simulink model "boat_model_and_controller2020mpc"  (R2020b)
settings: Solver=VariableStepAuto  StartTime=0.0  StopTime=10  FixedStep=0.01  RelTol=1e-3
undefined symbols (not defined in the file): DiscIntNeverNeededParam, Eff, FF_L, FF_R, initial_P, initial_Pitch, initial_Q, initial_R, initial_ROLL, initial_uspeed, initial_vspeed, initial_wspeed, initial_YAW, initial_Z, Kih, Kir, rear_alfas, T, uncertainty
libraries: simulink x7, simulink_extras x3, dspsrcs4 x1, mpclib x1, pid_lib x1
(part 1 of 3)
settings Model: Creator=Basile  LastModifiedBy=sasas
settings SolverCC: ConcurrentTasks=on  PositivePriorityOrder=on
settings DataIOCC: ExternalInput=getinputstruct(op_trim1)  InitialState=getstatestruct(op_trim1)  SaveOutput=off  DSMLogging=off  SaveTime=off  ReturnWorkspaceOutputs=off
settings OptimizationCC: BlockReduction=off  DefaultParameterBehavior=Inlined  UseDivisionForNetSlopeComputation=on  UseFloatMulNetSlope=on  OptimizeBlockIOStorage=off  BufferReuse=off  PassReuseOutputArgsThreshold=0  EfficientFloat2IntCast=on  OptimizeBlockOrder=speed  DifferentSizesBufferReuse=on
settings DebuggingCC: InheritedTsInSrcMsg=none  ParameterTunabilityLossMsg=error  UnconnectedInputMsg=none  UnconnectedOutputMsg=none  UnconnectedLineMsg=none  UniqueDataStoreMsg=error  ArithmeticOperatorsInVariantConditions=warning
settings HardwareCC: ProdBitPerLong=64  ProdLongLongMode=on  ProdHWDeviceType=Intel->x86-64 (Linux 64)
settings SFSimCC: SimUseLocalCustomCode=off  MATLABDynamicMemAlloc=off  CustomCodeUndefinedFunction=UseInterfaceOnly
settings RTWCC: Description=Simulink Real-Time  SystemTargetFile=slrealtime.tlc  TemplateMakefile=slrealtime_default_tmf  GenerateReport=on  RTWUseLocalCustomCode=off  Toolchain=Simulink Real-Time Toolchain  BuildConfiguration=Faster Runs  LaunchReport=on  CodeExecutionProfiling=on  TargetLang=C++
settings CodeAppCC: ForceParamTrailComments=on  OperatorAnnotations=on

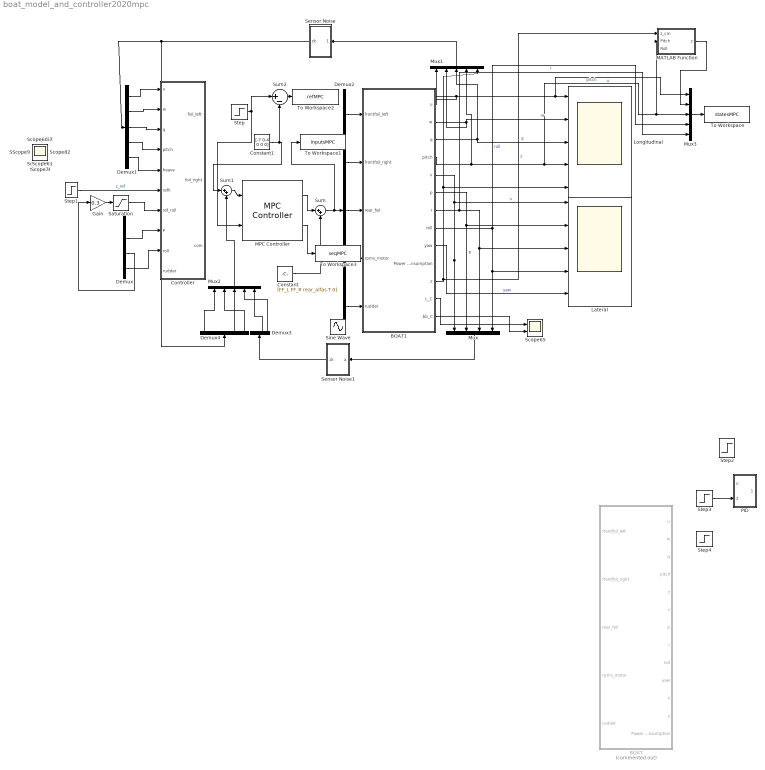
== system boat_model_and_controller2020mpc ==
  BOAT : Subsystem  Commented=on
  BOAT1 : Subsystem
  Constant : Constant  Value=[FF_L FF_R rear_alfas T 0]
  Constant1 : Constant  Value=[-7 0.4 0 0 0]
  Controller : Subsystem
  Demux : Demux
  Demux1 : Demux  Outputs=5
  Demux2 : Demux  Outputs=5
  Demux3 : Demux
  Demux4 : Demux  Outputs=5
  Gain : Gain  Gain=0.3
  Lateral : Scope  NumInputPorts=5
  Longitudinal : Scope  NumInputPorts=5
  MATLAB Function : MATLAB Function  TreatAsAtomicUnit=on
  MPC Controller : mpclib/MPC Controller  SCDEnableBlockLinearizationSpecification=on  mpcobj=mpcobj  x0=Boat_mpc  is_multiple=0  enable_value=0  return_u0=off  updateMPCinCallerWorkspace=on  md_inport=off  mv_inport=off  uref_inport=off  return_cost=off  return_mvseq=off  return_qpstatus=off  return_xseq=off  return_state=off  return_ovseq=on  state_inport=off  umin_inport=off  umax_inport=off  ymin_inport=off  ymax_inport=off  cc_inport=off  ywt_inport=off  uwt_inport=off  duwt_inport=off  rhoeps_inport=off  pm_inport=off  MaximumP=10  HorizonChoice=FixedHorizon  n_ts=0.1  n_p=20  n_mv=5  n_md=0  n_ud=0  n_mo=5  n_uo=0  BlockDataType=double  SampleTimeInherited=off  switch_inport=off
  Mux : Mux
  Mux1 : Mux  Inputs=5
  Mux2 : Mux  Inputs=5
  Mux3 : Mux  Inputs=5
  PID : Subsystem
  Saturation : Saturate  UpperLimit=3  LowerLimit=-3
  Scope65 : Scope  NumInputPorts=2
  Sensor Noise : Subsystem
  Sensor Noise1 : Subsystem
  Sine Wave : Sin  Amplitude=15  Frequency=0.1*2*pi  SampleTime=0
  Step : Step  Before=[0 0 0 0 0]  After=[1 -0.1 1 1 1]  SampleTime=0
  Step1 : Step  Time=0  Before=initial_Z  After=initial_Z  SampleTime=0
  Step2 : Step  Time=0  Before=rear_alfas  After=rear_alfas  SampleTime=0
  Step3 : Step  Time=10  Before=initial_uspeed  After=8  SampleTime=0
  Step4 : Step  Time=0  Before=15  After=15  SampleTime=0
  Sum : Sum  Inputs=|++
  Sum1 : Sum  Inputs=|++
  Sum2 : Sum  Inputs=|+-
  To Workspace : ToWorkspace  VariableName=statesMPC  SaveFormat=Timeseries  SampleTime=-1
  To Workspace1 : ToWorkspace  VariableName=inputsMPC  SaveFormat=Timeseries  SampleTime=-1
  To Workspace2 : ToWorkspace  VariableName=refMPC  SaveFormat=Timeseries  SampleTime=-1
  To Workspace3 : ToWorkspace  VariableName=seqMPC  SaveFormat=Timeseries  SampleTime=-1
  Scope{,1..64} (65 alike) : Scope
  wires:
  BOAT1/2(w) -> Longitudinal/2, Mux1/2  "w"
  BOAT1/3(q) -> Longitudinal/3, Mux1/3  "q"
  BOAT1/5(v) -> Mux/1, Lateral/1  "v"
  BOAT1/6(p) -> Mux/2, Lateral/2  "p"
  BOAT1/8(roll) -> Mux/4, Lateral/4, Mux3/4  "roll"
  BOAT1/11(z) -> MATLAB Function/1(z_cm), Mux1/5, Longitudinal/5  "z"
  BOAT1/1(u) -> Mux3/1, Longitudinal/1, Mux1/1  "u"
  BOAT1/7(r) -> Mux3/5, Mux/3, Lateral/3  "r"
  Demux/2 -> Controller/8(P)
  Demux1/2 -> Controller/2(w)
  Demux1/3 -> Controller/3(q)
  Demux1/4 -> Controller/4(pitch)
  Demux1/5 -> Controller/5(heave)
  Demux1/1 -> Controller/1(u)
  BOAT1/9(yaw) -> Lateral/5  "yaw"
  BOAT1/4(pitch) -> MATLAB Function/2(Pitch), Mux3/3, Longitudinal/4, Mux1/4  "pitch"
  Demux/4 -> Controller/9(roll)
  Mux1/1 -> Sensor Noise/1(states)
  Step1/1 -> Controller/6(refh)  "z_ref"
  Mux/1 -> Sensor Noise1/1(a)
  Step3/1 -> PID/2(In2)
  Gain/1 -> Saturation/1
  Saturation/1 -> Controller/7(ref_roll)
  Demux/3 -> Gain/1
  BOAT1/12(L_C) -> Scope65/1
  BOAT1/13(bb_C) -> Scope65/2
  Demux2/1 -> BOAT1/1(frontfoil_left)
  Demux2/2 -> BOAT1/2(frontfoil_right)
  Demux2/3 -> BOAT1/3(rear_foil)
  Demux2/4 -> BOAT1/4(rpms_motor)
  Demux2/5 -> BOAT1/5(rudder)
  MPC Controller/1 -> Sum/1
  Sensor Noise1/1(zk) -> Demux3/1
  Demux4/1 -> Mux2/1
  Demux4/5 -> Mux2/2
  Demux4/4 -> Mux2/3
  Demux3/4 -> Mux2/4
  Demux3/3 -> Mux2/5
  Sum1/1 -> MPC Controller/1
  Mux2/1 -> Sum1/2
  Constant1/1 -> Sum1/1, Sum2/2
  Step/1 -> MPC Controller/2, Sum2/1
  Sensor Noise/1(zk) -> Demux1/1, Demux4/1
  Sum/1 -> To Workspace1/1, Demux2/1
  Constant/1 -> Sum/2
  Mux3/1 -> To Workspace/1
  Sum2/1 -> To Workspace2/1
  MATLAB Function/1(z) -> Mux3/2
  MPC Controller/2 -> To Workspace3/1

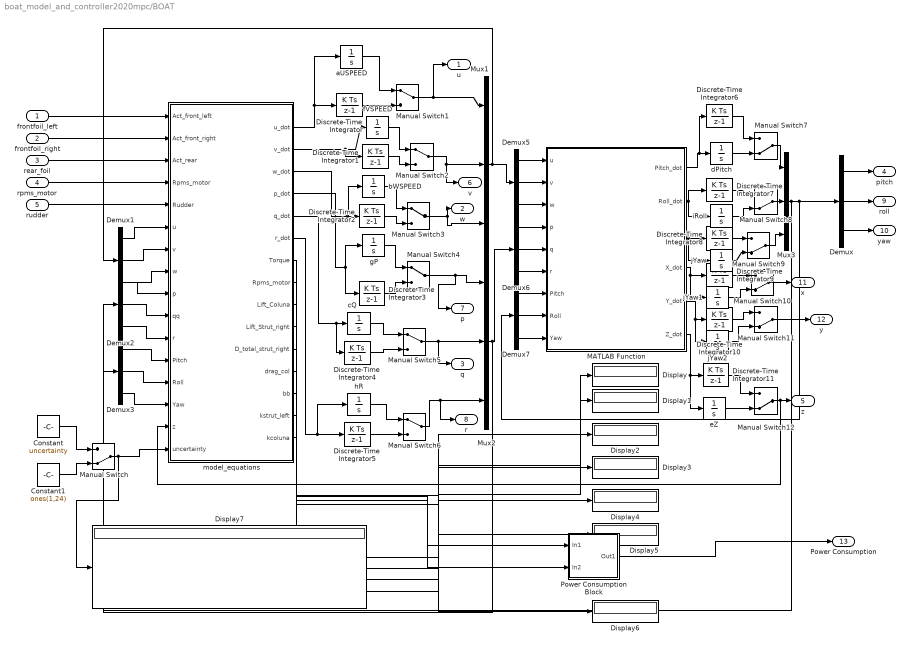
== system boat_model_and_controller2020mpc/BOAT ==
  frontfoil_left : Inport
  frontfoil_right : Inport  Port=2
  rear_foil : Inport  Port=3
  rpms_motor : Inport  Port=4
  rudder : Inport  Port=5
  Constant : Constant  Value=uncertainty
  Constant1 : Constant  Value=ones(1,24)
  Demux{,1..3,5..7} (7 alike) : Demux  Outputs=3
  Discrete-Time Integrator : DiscreteIntegrator  InitialCondition=initial_uspeed  SampleTime=-1  ICPrevOutput=DiscIntNeverNeededParam  ICPrevScaledInput=DiscIntNeverNeededParam
  Discrete-Time Integrator{1..10} (10 alike) : DiscreteIntegrator  SampleTime=-1  ICPrevOutput=DiscIntNeverNeededParam  ICPrevScaledInput=DiscIntNeverNeededParam
  Discrete-Time Integrator11 : DiscreteIntegrator  InitialCondition=initial_Z  SampleTime=-1  ICPrevOutput=DiscIntNeverNeededParam  ICPrevScaledInput=DiscIntNeverNeededParam
  Display{,1..7} (8 alike) : Display
  MATLAB Function : MATLAB Function  TreatAsAtomicUnit=on
  Manual Switch{,7..12} (7 alike) : ManualSwitch  CurrentSetting=0
  Manual Switch{1..6} (6 alike) : ManualSwitch
  Mux1 : Mux  Inputs=3
  Mux2 : Mux  Inputs=3
  Mux3 : Mux  Inputs=3
  Power Consumption Block : Subsystem
  aUSPEED : Integrator  InitialCondition=initial_uspeed
  bWSPEED : Integrator  InitialCondition=initial_wspeed
  cQ : Integrator  InitialCondition=initial_Q
  dPitch : Integrator  InitialCondition=initial_Pitch
  eZ : Integrator  InitialCondition=initial_Z
  fVSPEED : Integrator  InitialCondition=initial_vspeed
  gP : Integrator  InitialCondition=initial_P
  hR : Integrator  InitialCondition=initial_R
  iRoll : Integrator  InitialCondition=initial_ROLL
  jYaw : Integrator  InitialCondition=initial_YAW
  jYaw1 : Integrator
  jYaw2 : Integrator
  model_equations : MATLAB Function  TreatAsAtomicUnit=on  VariantControl=Variant1
  u : Outport  VectorParamsAs1DForOutWhenUnconnected=off
  w : Outport  Port=2  VectorParamsAs1DForOutWhenUnconnected=off
  q : Outport  Port=3  VectorParamsAs1DForOutWhenUnconnected=off
  pitch : Outport  Port=4  VectorParamsAs1DForOutWhenUnconnected=off
  z : Outport  Port=5  VectorParamsAs1DForOutWhenUnconnected=off
  v : Outport  Port=6  VectorParamsAs1DForOutWhenUnconnected=off
  p : Outport  Port=7  VectorParamsAs1DForOutWhenUnconnected=off
  r : Outport  Port=8  VectorParamsAs1DForOutWhenUnconnected=off
  roll : Outport  Port=9  VectorParamsAs1DForOutWhenUnconnected=off
  yaw : Outport  Port=10  VectorParamsAs1DForOutWhenUnconnected=off
  x : Outport  Port=11  VectorParamsAs1DForOutWhenUnconnected=off
  y : Outport  Port=12  VectorParamsAs1DForOutWhenUnconnected=off
  Power Consumption : Outport  Port=13  VectorParamsAs1DForOutWhenUnconnected=off
  wires:
  model_equations/6(r_dot) -> hR/1, Discrete-Time Integrator5/1
  Demux5/3 -> MATLAB Function/3(w)
  frontfoil_left/1 -> model_equations/1(Act_front_left)
  frontfoil_right/1 -> model_equations/2(Act_front_right)
  Mux1/1 -> Demux5/1, Demux1/1
  Demux/2 -> roll/1
  Demux7/2 -> MATLAB Function/8(Roll)
  Demux7/3 -> MATLAB Function/9(Yaw)
  model_equations/5(q_dot) -> Discrete-Time Integrator4/1, cQ/1
  rear_foil/1 -> model_equations/3(Act_rear)
  model_equations/3(w_dot) -> bWSPEED/1, Discrete-Time Integrator2/1
  Demux3/2 -> model_equations/13(Roll)
  Demux2/2 -> model_equations/10(qq)
  Demux2/3 -> model_equations/11(r)
  model_equations/4(p_dot) -> Discrete-Time Integrator3/1, gP/1
  Demux2/1 -> model_equations/9(p)
  Demux5/1 -> MATLAB Function/1(u)
  rpms_motor/1 -> model_equations/4("Rpms_motor ")
  MATLAB Function/2(Roll_dot) -> iRoll/1, Discrete-Time Integrator7/1
  Demux7/1 -> MATLAB Function/7(Pitch)
  Mux3/1 -> Demux/1, Demux7/1, Demux3/1
  Demux3/1 -> model_equations/12(Pitch)
  model_equations/2(v_dot) -> fVSPEED/1, Discrete-Time Integrator1/1
  Demux/1 -> pitch/1
  Demux1/2 -> model_equations/7(v)
  Demux6/1 -> MATLAB Function/4(p)
  MATLAB Function/1(Pitch_dot) -> Discrete-Time Integrator6/1, dPitch/1
  Mux2/1 -> Demux6/1, Demux2/1
  Demux5/2 -> MATLAB Function/2(v)
  Demux/3 -> yaw/1
  rudder/1 -> model_equations/5(Rudder)
  Demux6/2 -> MATLAB Function/5(q)
  Demux1/3 -> model_equations/8(w)
  Demux6/3 -> MATLAB Function/6(r)
  Demux3/3 -> model_equations/14(Yaw)
  MATLAB Function/5(Y_dot) -> Discrete-Time Integrator10/1, jYaw2/1
  MATLAB Function/4(X_dot) -> Discrete-Time Integrator9/1, jYaw1/1
  model_equations/8(Rpms_motor) -> Power Consumption Block/2(In2)
  Power Consumption Block/1(Out1) -> Power Consumption/1
  model_equations/7(Torque) -> Power Consumption Block/1(In1)
  model_equations/9(Lift_Coluna) -> Display/1
  model_equations/10(Lift_Strut_right) -> Display1/1
  model_equations/11(D_total_strut_right) -> Display2/1
  model_equations/12(drag_col) -> Display3/1
  model_equations/13(bb) -> Display4/1
  model_equations/14(kstrut_left) -> Display5/1
  model_equations/15(kcoluna) -> Display6/1
  Demux1/1 -> model_equations/6(u)
  Constant/1 -> Manual Switch/1
  Manual Switch/1 -> model_equations/16(uncertainty), Display7/1
  Constant1/1 -> Manual Switch/2
  Discrete-Time Integrator/1 -> Manual Switch1/2
  Manual Switch1/1 -> Mux1/1, u/1
  aUSPEED/1 -> Manual Switch1/1
  fVSPEED/1 -> Manual Switch2/1
  Manual Switch2/1 -> v/1, Mux1/2
  bWSPEED/1 -> Manual Switch3/1
  Manual Switch3/1 -> Mux1/3, w/1
  gP/1 -> Manual Switch4/1
  Manual Switch4/1 -> Mux2/1, p/1
  cQ/1 -> Manual Switch5/1
  Manual Switch5/1 -> Mux2/2, q/1
  Manual Switch6/1 -> r/1, Mux2/3
  hR/1 -> Manual Switch6/1
  Discrete-Time Integrator1/1 -> Manual Switch2/2
  Discrete-Time Integrator2/1 -> Manual Switch3/2
  Discrete-Time Integrator3/1 -> Manual Switch4/2
  Discrete-Time Integrator4/1 -> Manual Switch5/2
  Discrete-Time Integrator5/1 -> Manual Switch6/2
  Manual Switch7/1 -> Mux3/1
  dPitch/1 -> Manual Switch7/2
  Discrete-Time Integrator6/1 -> Manual Switch7/1
  Manual Switch8/1 -> Mux3/2
  iRoll/1 -> Manual Switch8/2
  Discrete-Time Integrator7/1 -> Manual Switch8/1
  Manual Switch9/1 -> Mux3/3
  jYaw/1 -> Manual Switch9/2
  Discrete-Time Integrator8/1 -> Manual Switch9/1
  MATLAB Function/3(Yaw_dot) -> Discrete-Time Integrator8/1, jYaw/1
  Manual Switch10/1 -> x/1
  jYaw1/1 -> Manual Switch10/2
  Discrete-Time Integrator9/1 -> Manual Switch10/1
  Manual Switch11/1 -> y/1
  Discrete-Time Integrator10/1 -> Manual Switch11/1
  jYaw2/1 -> Manual Switch11/2
  Manual Switch12/1 -> model_equations/15(z), z/1
  eZ/1 -> Manual Switch12/2
  Discrete-Time Integrator11/1 -> Manual Switch12/1
  MATLAB Function/6(Z_dot) -> eZ/1, Discrete-Time Integrator11/1
  model_equations/1(u_dot) -> aUSPEED/1, Discrete-Time Integrator/1

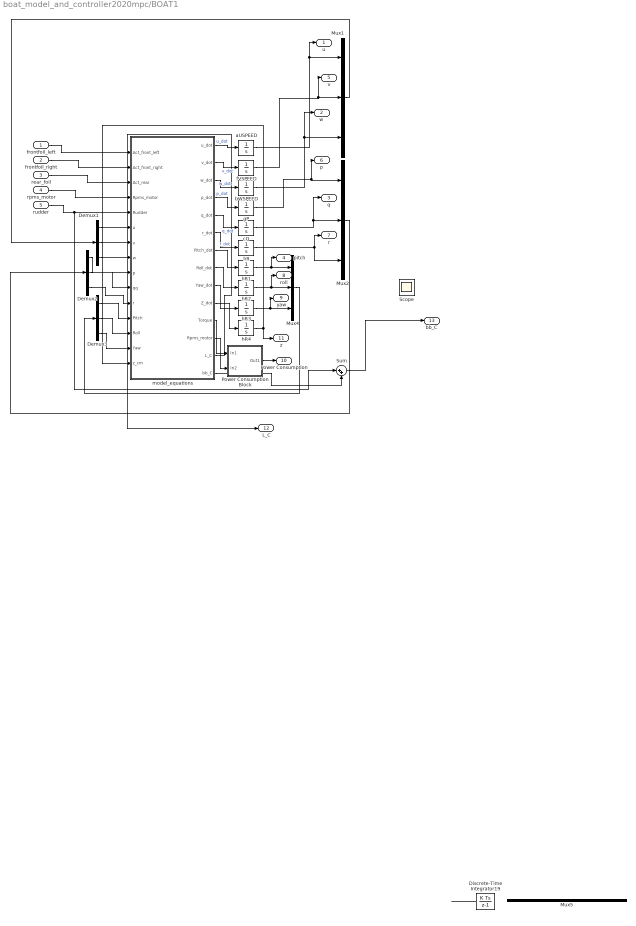
== system boat_model_and_controller2020mpc/BOAT1 ==
  frontfoil_left : Inport
  frontfoil_right : Inport  Port=2
  rear_foil : Inport  Port=3
  rpms_motor : Inport  Port=4
  rudder : Inport  Port=5
  Demux1 : Demux  Outputs=3
  Demux2 : Demux  Outputs=3
  Demux3 : Demux  Outputs=3
  Discrete-Time Integrator19 : DiscreteIntegrator  InitialCondition=-0.4  SampleTime=-1  ICPrevOutput=DiscIntNeverNeededParam  ICPrevScaledInput=DiscIntNeverNeededParam
  Mux{1..2,4..5} (4 alike) : Mux  Inputs=3
  Power Consumption Block : Subsystem
  Scope : Scope
  Sum : Sum  Inputs=|++
  aUSPEED : Integrator  InitialCondition=initial_uspeed
  bWSPEED : Integrator  InitialCondition=initial_wspeed
  cQ : Integrator  InitialCondition=initial_Q
  fVSPEED : Integrator  InitialCondition=initial_vspeed
  gP : Integrator  InitialCondition=initial_P
  hR : Integrator  InitialCondition=initial_R
  hR1 : Integrator
  hR2 : Integrator
  hR3 : Integrator
  hR4 : Integrator  InitialCondition=initial_Z
  model_equations : MATLAB Function  TreatAsAtomicUnit=on  VariantControl=Variant1
  u : Outport  VectorParamsAs1DForOutWhenUnconnected=off
  w : Outport  Port=2  VectorParamsAs1DForOutWhenUnconnected=off
  q : Outport  Port=3  VectorParamsAs1DForOutWhenUnconnected=off
  pitch : Outport  Port=4  VectorParamsAs1DForOutWhenUnconnected=off
  v : Outport  Port=5  VectorParamsAs1DForOutWhenUnconnected=off
  p : Outport  Port=6  VectorParamsAs1DForOutWhenUnconnected=off
  r : Outport  Port=7  VectorParamsAs1DForOutWhenUnconnected=off
  roll : Outport  Port=8  VectorParamsAs1DForOutWhenUnconnected=off
  yaw : Outport  Port=9  VectorParamsAs1DForOutWhenUnconnected=off
  Power Consumption : Outport  Port=10  VectorParamsAs1DForOutWhenUnconnected=off
  z : Outport  Port=11  VectorParamsAs1DForOutWhenUnconnected=off
  L_C : Outport  Port=12  VectorParamsAs1DForOutWhenUnconnected=off
  bb_C : Outport  Port=13  VectorParamsAs1DForOutWhenUnconnected=off
  wires:
  model_equations/6(r_dot) -> hR/1  "r_dot"
  Mux1/1 -> Demux1/1
  model_equations/5(q_dot) -> cQ/1  "q_dot"
  rear_foil/1 -> model_equations/3(Act_rear)
  Demux3/2 -> model_equations/13(Roll)
  Demux2/2 -> model_equations/10(qq)
  Demux2/3 -> model_equations/11(r)
  model_equations/4(p_dot) -> gP/1  "p_dot"
  Demux2/1 -> model_equations/9(p)
  rpms_motor/1 -> model_equations/4("Rpms_motor ")
  Demux3/1 -> model_equations/12(Pitch)
  model_equations/2(v_dot) -> fVSPEED/1  "v_dot"
  Demux1/2 -> model_equations/7(v)
  Mux2/1 -> Demux2/1
  Demux1/3 -> model_equations/8(w)
  Demux3/3 -> model_equations/14(Yaw)
  model_equations/12(Rpms_motor) -> Power Consumption Block/2(In2)
  Power Consumption Block/1(Out1) -> Power Consumption/1
  model_equations/11(Torque) -> Power Consumption Block/1(In1)
  Demux1/1 -> model_equations/6(u)
  aUSPEED/1 -> u/1, Mux1/1
  fVSPEED/1 -> v/1, Mux1/2
  cQ/1 -> q/1, Mux2/2
  hR/1 -> Mux2/3, r/1
  model_equations/3(w_dot) -> bWSPEED/1  "w_dot"
  model_equations/1(u_dot) -> aUSPEED/1  "u_dot"
  Discrete-Time Integrator19/1 -> ?
  bWSPEED/1 -> w/1, Mux1/3
  gP/1 -> p/1, Mux2/1
  model_equations/10(Z_dot) -> hR4/1
  model_equations/7(Pitch_dot) -> hR1/1
  model_equations/8(Roll_dot) -> hR2/1
  model_equations/9(Yaw_dot) -> hR3/1
  hR1/1 -> pitch/1, Mux4/1
  hR2/1 -> roll/1, Mux4/2
  hR3/1 -> yaw/1, Mux4/3
  Mux4/1 -> Demux3/1
  hR4/1 -> z/1, model_equations/15(z_cm)
  model_equations/13(L_C) -> L_C/1
  rudder/1 -> Sum/1, model_equations/5(Rudder)
  model_equations/14(bb_C) -> Sum/2
  Sum/1 -> bb_C/1
  frontfoil_left/1 -> model_equations/1(Act_front_left)
  frontfoil_right/1 -> model_equations/2(Act_front_right)

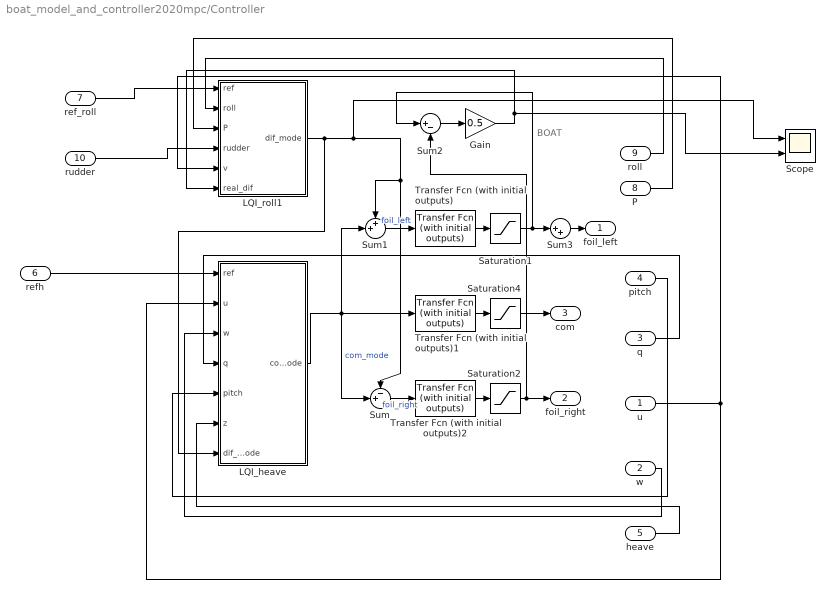
== system boat_model_and_controller2020mpc/Controller ==
  note: BOAT
  u : Inport
  w : Inport  Port=2
  q : Inport  Port=3
  pitch : Inport  Port=4
  heave : Inport  Port=5
  refh : Inport  Port=6
  ref_roll : Inport  Port=7
  P : Inport  Port=8
  roll : Inport  Port=9
  rudder : Inport  Port=10
  Gain : Gain  Gain=0.5
  LQI_heave : Subsystem  TreatAsAtomicUnit=on  SystemSampleTime=0.02
      settings: MinAlgLoopOccurrences=on
  LQI_roll1 : Subsystem  TreatAsAtomicUnit=on  SystemSampleTime=0.02
  Saturation1 : Saturate  UpperLimit=14  LowerLimit=-3
  Saturation2 : Saturate  UpperLimit=14  LowerLimit=-3
  Saturation4 : Saturate  UpperLimit=14  LowerLimit=-3
  Scope : Scope  NumInputPorts=2
  Sum : Sum  Inputs=-+|
  Sum1 : Sum  Inputs=++|
  Sum2 : Sum  Inputs=|+-
  Sum3 : Sum  Inputs=|++
  Transfer Fcn (with initial outputs) : simulink_extras/Additional Linear/Transfer Fcn (with initial outputs)  N=[40]  D="[1  40]"  Y0=FF_L  U0=FF_L
  Transfer Fcn (with initial outputs)1 : simulink_extras/Additional Linear/Transfer Fcn (with initial outputs)  N=[40]  D="[1  40]"  Y0=(FF_L+FF_R)/2  U0=(FF_L+FF_R)/2
  Transfer Fcn (with initial outputs)2 : simulink_extras/Additional Linear/Transfer Fcn (with initial outputs)  N=[40]  D="[1  40]"  Y0=FF_R  U0=FF_R
  foil_left : Outport  VectorParamsAs1DForOutWhenUnconnected=off
  foil_right : Outport  Port=2  VectorParamsAs1DForOutWhenUnconnected=off
  com : Outport  Port=3  VectorParamsAs1DForOutWhenUnconnected=off
  wires:
  LQI_heave/1(com_mode) -> Sum/2, Transfer Fcn (with initial outputs)1/1, Sum1/2  "com_mode"
  roll/1 -> LQI_roll1/2(roll)
  pitch/1 -> LQI_heave/5(pitch)
  u/1 -> LQI_roll1/5(v), LQI_heave/2(u)
  w/1 -> LQI_heave/3(w)
  P/1 -> LQI_roll1/3(P)
  heave/1 -> LQI_heave/6(z)
  refh/1 -> LQI_heave/1(ref)
  Saturation1/1 -> Sum3/1, Sum2/1
  Saturation2/1 -> Sum2/2, foil_right/1
  Saturation4/1 -> com/1
  ref_roll/1 -> LQI_roll1/1(ref)
  LQI_roll1/1(dif_mode) -> LQI_heave/7(dif_mode), Scope/1, Sum/1, Sum1/1
  rudder/1 -> LQI_roll1/4(rudder)
  q/1 -> LQI_heave/4(q)
  Transfer Fcn (with initial outputs)1/1 -> Saturation4/1
  Transfer Fcn (with initial outputs)/1 -> Saturation1/1
  Sum1/1 -> Transfer Fcn (with initial outputs)/1  "foil_left"
  Sum/1 -> Transfer Fcn (with initial outputs)2/1  "foil_right"
  Transfer Fcn (with initial outputs)2/1 -> Saturation2/1
  Gain/1 -> Scope/2, LQI_roll1/6(real_dif)
  Sum2/1 -> Gain/1
  Sum3/1 -> foil_left/1

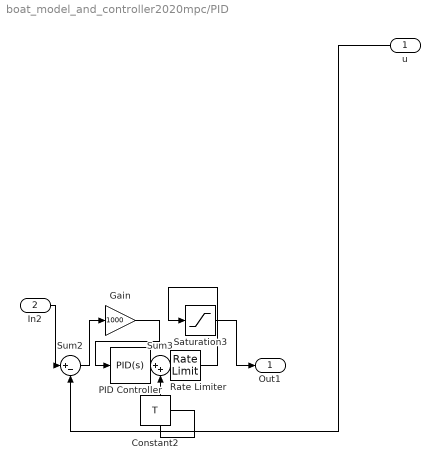
== system boat_model_and_controller2020mpc/PID ==
  u : Inport
  In2 : Inport  Port=2
  Constant2 : Constant  Value=T
  Gain : Gain  Gain=1000
  PID Controller : pid_lib/PID Controller  Controller=PID  Form=Parallel  TimeDomain=Continuous-time  UseExternalTs=off  SampleTime=-1  IntegratorMethod=Forward Euler  FilterMethod=Forward Euler  ControllerParametersSource=internal  P=1  I=1  D=0.00001  UseFilter=on  N=100  TunerSelectOption=Transfer Function Based (PID Tuner App)  InitialConditionSource=internal  InitialConditionForIntegrator=0  InitialConditionForFilter=0  DifferentiatorICPrevScaledInput=0  ExternalReset=none  TrackingMode=off  Kt=1  LimitOutput=off  SatLimitsSource=internal  UpperSaturationLimit=inf  LowerSaturationLimit=-inf  LinearizeAsGain=on  AntiWindupMode=none  Kb=1  POutMin=[]  POutMax=[]  IOutMin=[]  IOutMax=[]  DOutMin=[]  DOutMax=[]  NOutMin=[]  NOutMax=[]  SumOutMin=[]  SumOutMax=[]  SaturationOutMin=[]  SaturationOutMax=[]  PParamMin=[]  PParamMax=[]  IParamMin=[]  IParamMax=[]  DParamMin=[]  DParamMax=[]  NParamMin=[]  NParamMax=[]  KbParamMin=[]  KbParamMax=[]  KtParamMin=[]  KtParamMax=[]  KbOutMin=[]  KbOutMax=[]  KtOutMin=[]  KtOutMax=[]  IntegratorOutMin=[]  IntegratorOutMax=[]  FilterOutMin=[]  FilterOutMax=[]  SumI1OutMin=[]  SumI1OutMax=[]  SumI2OutMin=[]  SumI2OutMax=[]  SumI3OutMin=[]  SumI3OutMax=[]  SumI4OutMin=[]  SumI4OutMax=[]  SumDOutMin=[]  SumDOutMax=[]  DifferentiatorOutMin=[]  DifferentiatorOutMax=[]  FilterDiffOutCoefMin=[]  FilterDiffOutCoefMax=[]  ReciprocalOutMin=[]  ReciprocalOutMax=[]  SumDenOutMin=[]  SumDenOutMax=[]  SumNumOutMin=[]  SumNumOutMax=[]  DivideOutMin=[]  DivideOutMax=[]  UdiffTsProdOutMin=[]  UdiffTsProdOutMax=[]  NTsProdOutMin=[]  NTsProdOutMax=[]  UintegralTsProdOutMin=[]  UintegralTsProdOutMax=[]  UngainTsProdOutMin=[]  UngainTsProdOutMax=[]  IntegratorContinuousStateAttributes=''  IntegratorStateMustResolveToSignalObject=off  IntegratorRTWStateStorageClass=Auto  FilterContinuousStateAttributes=''  FilterStateMustResolveToSignalObject=off  FilterRTWStateStorageClass=Auto  ParallelPVariant=InternalParameters  IdealPVariant=Disabled  IVariant=InternalParameters  DVariant=InternalParameters  IntegratorVariant=Continuous  SatVariant=Disabled  AWVariant=Passthrough  PCopyVariant=Disabled  TRVariant=Disabled  FdbkBlocksVariant=Forward  IdealPFdbkVariant=Disabled  SatFdbkVariant=Disabled  DerivativeFilterVariant=ContFilter  NVariant=InternalParameters  NCopyVariant=Disabled  FilterICVariant=InternalICsFilter  IntegratorICVariant=InternalICs  ExternalResetVariant=Disabled  TRSumVariant=Passthrough  SumFdbkVariant=Disabled  SumVariant=Sum_PID  TsampFilterVariant=InternalTs  TsampNgainVariant=Passthrough  TsampIntegralVariant=Passthrough  ExternalSaturationOutDataTypeStr=Inherit: Same as second input
  Rate Limiter : RateLimiter  RisingSlewLimit=1000  FallingSlewLimit=-1000  SampleTimeMode=inherited  InitialCondition=T
  Saturation3 : Saturate  UpperLimit=6000
  Sum2 : Sum  Inputs=|+-
  Sum3 : Sum  Inputs=|++
  Out1 : Outport
  wires:
  u/1 -> Sum2/2
  Sum3/1 -> Rate Limiter/1
  Gain/1 -> PID Controller/1
  Saturation3/1 -> Out1/1
  PID Controller/1 -> Sum3/1
  Rate Limiter/1 -> Saturation3/1
  Sum2/1 -> Gain/1
  In2/1 -> Sum2/1
  Constant2/1 -> Sum3/2

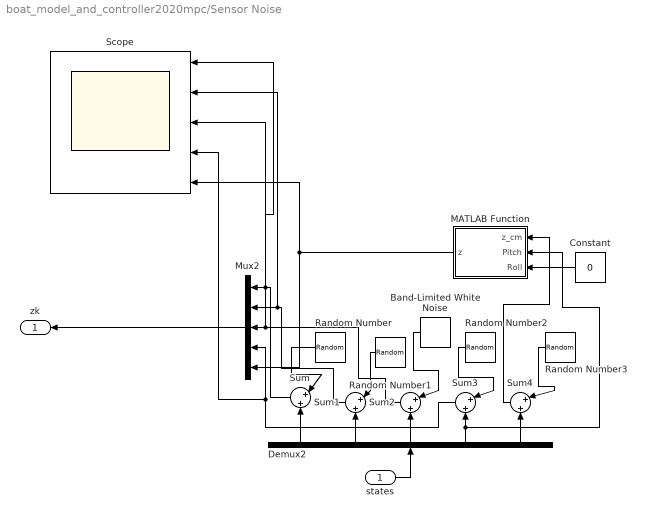
== system boat_model_and_controller2020mpc/Sensor Noise ==
  states : Inport
  Band-Limited White Noise : simulink/Sources/Band-Limited White Noise  Cov=15*[0.01^2]  Ts=0.02  seed=[23341]
  Constant : Constant  Value=0
  Demux2 : Demux  Outputs=5
  MATLAB Function : MATLAB Function  TreatAsAtomicUnit=on
  Mux2 : Mux  Inputs=5
  Random Number : RandomNumber  Variance=2*0.05^2  Seed=31233  SampleTime=0.02
  Random Number1 : RandomNumber  Variance=2*0.05^2  Seed=31232  SampleTime=0.02
  Random Number2 : RandomNumber  Variance=1*0.25^2  Seed=372323  SampleTime=0.02
  Random Number3 : RandomNumber  Variance=2*0.005^2  Seed=312392  SampleTime=0.02
  Scope : Scope  NumInputPorts=5
  Sum{,1..4} (5 alike) : Sum  Inputs=|+|+
  zk : Outport
  wires:
  Sum2/1 -> Scope/3, Mux2/3
  Demux2/1 -> Sum/2
  Random Number2/1 -> Sum3/1
  Random Number3/1 -> Sum4/1
  Random Number/1 -> Sum/1
  Demux2/4 -> MATLAB Function/2(Pitch), Sum3/2
  Demux2/3 -> Sum2/2
  Demux2/5 -> Sum4/2
  Demux2/2 -> Sum1/2
  Random Number1/1 -> Sum1/1
  Sum/1 -> Scope/1, Mux2/1
  Sum1/1 -> Scope/2, Mux2/2
  Sum3/1 -> Mux2/4, Scope/4
  states/1 -> Demux2/1
  Mux2/1 -> zk/1
  Band-Limited White Noise/1 -> Sum2/1
  Sum4/1 -> MATLAB Function/1(z_cm)
  Constant/1 -> MATLAB Function/3(Roll)
  MATLAB Function/1(z) -> Mux2/5, Scope/5

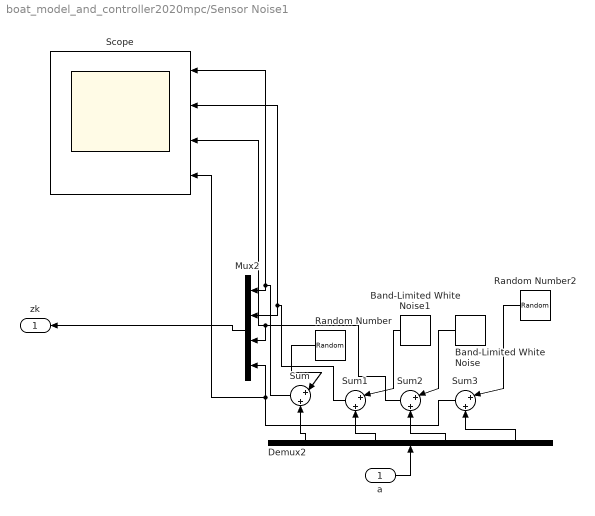
== system boat_model_and_controller2020mpc/Sensor Noise1 ==
  a : Inport
  Band-Limited White Noise : simulink/Sources/Band-Limited White Noise  Cov=15*[0.01^2]  Ts=0.02  seed=[23341]
  Band-Limited White Noise1 : simulink/Sources/Band-Limited White Noise  Cov=15*[0.01^2]  Ts=0.02  seed=[23371]
  Demux2 : Demux
  Mux2 : Mux
  Random Number : RandomNumber  Variance=2*0.05^2  Seed=31233  SampleTime=0.02
  Random Number2 : RandomNumber  Variance=1*0.25^2  Seed=372323  SampleTime=0.02
  Scope : Scope  NumInputPorts=4
  Sum{,1..3} (4 alike) : Sum  Inputs=|+|+
  zk : Outport
  wires:
  Sum2/1 -> Scope/3, Mux2/3
  Demux2/1 -> Sum/2
  Random Number/1 -> Sum/1
  Demux2/4 -> Sum3/2
  Demux2/3 -> Sum2/2
  Demux2/2 -> Sum1/2
  Sum/1 -> Scope/1, Mux2/1
  Sum1/1 -> Scope/2, Mux2/2
  Sum3/1 -> Mux2/4, Scope/4
  a/1 -> Demux2/1
  Mux2/1 -> zk/1
  Band-Limited White Noise/1 -> Sum2/1
  Random Number2/1 -> Sum3/1
  Band-Limited White Noise1/1 -> Sum1/1

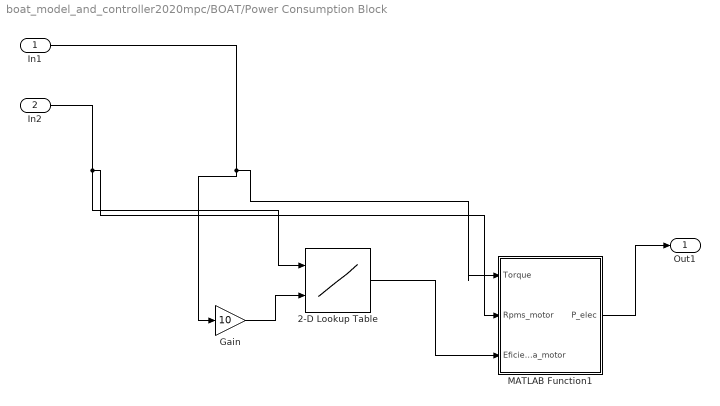
== system boat_model_and_controller2020mpc/BOAT/Power Consumption Block ==
  In1 : Inport
  In2 : Inport  Port=2
  2-D Lookup Table : Lookup_n-D  BreakpointsForDimension1=[1:6000]  BreakpointsForDimension2=[1:140]  Table=Eff  InternalRulePriority=Speed  RndMeth=Simplest  InputSameDT=on
      settings: InputPortMap=u0,u1
  Gain : Gain  Gain=10
  MATLAB Function1 : MATLAB Function  TreatAsAtomicUnit=on
  Out1 : Outport
  wires:
  In2/1 -> 2-D Lookup Table/1, MATLAB Function1/2(Rpms_motor)
  MATLAB Function1/1(P_elec) -> Out1/1
  In1/1 -> Gain/1, MATLAB Function1/1(Torque)
  Gain/1 -> 2-D Lookup Table/2
  2-D Lookup Table/1 -> MATLAB Function1/3(Eficiencia_motor)

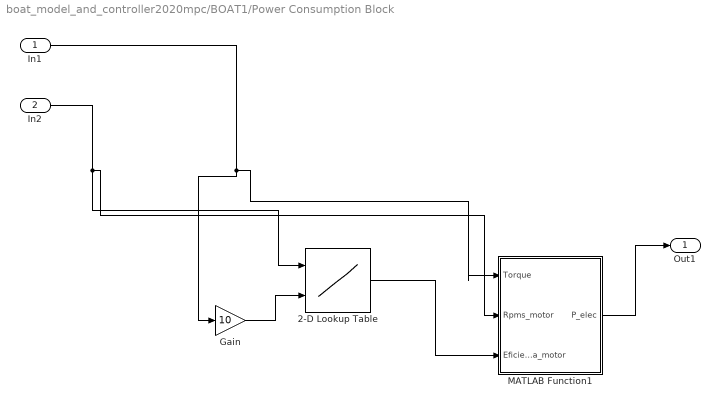
== system boat_model_and_controller2020mpc/BOAT1/Power Consumption Block ==
  In1 : Inport
  In2 : Inport  Port=2
  2-D Lookup Table : Lookup_n-D  BreakpointsForDimension1=[1:6000]  BreakpointsForDimension2=[1:140]  Table=Eff  InternalRulePriority=Speed  RndMeth=Simplest  InputSameDT=on
      settings: InputPortMap=u0,u1
  Gain : Gain  Gain=10
  MATLAB Function1 : MATLAB Function  TreatAsAtomicUnit=on
  Out1 : Outport
  wires:
  In2/1 -> 2-D Lookup Table/1, MATLAB Function1/2(Rpms_motor)
  MATLAB Function1/1(P_elec) -> Out1/1
  In1/1 -> Gain/1, MATLAB Function1/1(Torque)
  Gain/1 -> 2-D Lookup Table/2
  2-D Lookup Table/1 -> MATLAB Function1/3(Eficiencia_motor)

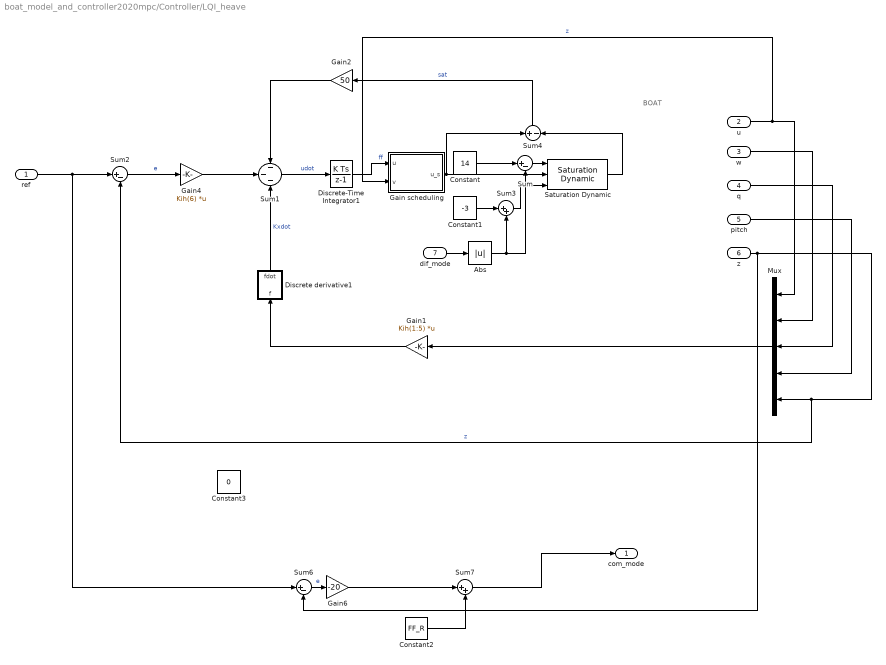
== system boat_model_and_controller2020mpc/Controller/LQI_heave ==
  note: BOAT
  ref : Inport
  u : Inport  Port=2
  w : Inport  Port=3
  q : Inport  Port=4
  pitch : Inport  Port=5
  z : Inport  Port=6
  dif_mode : Inport  Port=7
  Abs : Abs
  Constant : Constant  Value=14
  Constant1 : Constant  Value=-3
  Constant2 : Constant  Value=FF_R
  Constant3 : Constant  Value=0
  Discrete derivative1 : Subsystem
  Discrete-Time Integrator1 : DiscreteIntegrator  gainval=1  InitialCondition=FF_R  SampleTime=-1  ICPrevOutput=DiscIntNeverNeededParam  ICPrevScaledInput=DiscIntNeverNeededParam
  Gain scheduling : MATLAB Function  TreatAsAtomicUnit=on
  Gain1 : Gain  Gain=Kih(1:5)  Multiplication=Matrix(K*u)
  Gain2 : Gain  Gain=50
  Gain4 : Gain  Gain=Kih(6)  Multiplication=Matrix(K*u)
  Gain6 : Gain  Gain=-20
  Mux : Mux  Inputs=5
  Saturation Dynamic : simulink/Discontinuities/Saturation Dynamic  OutMin=[]  OutMax=[]  OutDataTypeStr=Inherit: Same as second input  OutDataType=fixdt(1, 16)  OutScaling=2^-10  DoSatur=off
  Sum : Sum  Inputs=|+-
  Sum1 : Sum  Inputs=---
  Sum2 : Sum  Inputs=|+-
  Sum3 : Sum  Inputs=|++
  Sum4 : Sum  Inputs=+|-
  Sum6 : Sum  Inputs=|+-
  Sum7 : Sum  Inputs=|++
  com_mode : Outport  VectorParamsAs1DForOutWhenUnconnected=off
  wires:
  Sum4/1 -> Gain2/1  "sat"
  Gain2/1 -> Sum1/1
  Sum1/1 -> Discrete-Time Integrator1/1  "udot"
  w/1 -> Mux/2
  q/1 -> Mux/3
  pitch/1 -> Mux/4
  u/1 -> Gain scheduling/2(v), Mux/1  "z"
  z/1 -> Mux/5, Sum2/2, Sum6/2  "z"
  Gain1/1 -> Discrete derivative1/1(f)
  Mux/1 -> Gain1/1
  Discrete derivative1/1(fdot) -> Sum1/3  "Kxdot"
  Gain4/1 -> Sum1/2
  Sum2/1 -> Gain4/1  "e"
  Discrete-Time Integrator1/1 -> Gain scheduling/1(u)  "ff"
  Gain scheduling/1(u_s) -> Saturation Dynamic/2, Sum4/1
  Sum/1 -> Saturation Dynamic/1
  Constant/1 -> Sum/1
  dif_mode/1 -> Abs/1
  Abs/1 -> Sum/2, Sum3/2
  Sum3/1 -> Saturation Dynamic/3
  Constant1/1 -> Sum3/1
  ref/1 -> Sum6/1, Sum2/1
  Constant2/1 -> Sum7/2
  Saturation Dynamic/1 -> Sum4/2
  Sum7/1 -> com_mode/1
  Gain6/1 -> Sum7/1
  Sum6/1 -> Gain6/1  "e"

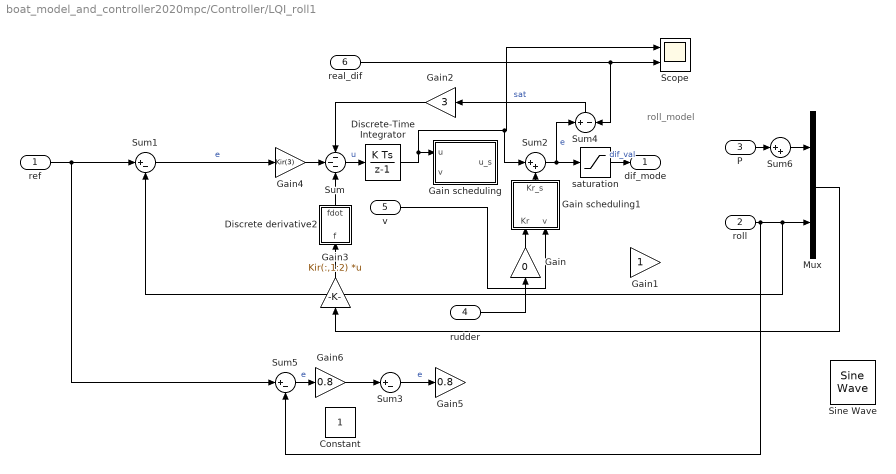
== system boat_model_and_controller2020mpc/Controller/LQI_roll1 ==
  note: roll_model
  ref : Inport
  roll : Inport  Port=2
  P : Inport  Port=3
  rudder : Inport  Port=4
  v : Inport  Port=5
  real_dif : Inport  Port=6
  Constant : Constant
  Discrete derivative2 : Subsystem
  Discrete-Time Integrator : DiscreteIntegrator  gainval=1  SampleTime=-1  ICPrevOutput=DiscIntNeverNeededParam  ICPrevScaledInput=DiscIntNeverNeededParam
  Gain : Gain  Gain=0
  Gain scheduling : MATLAB Function  TreatAsAtomicUnit=on
  Gain scheduling1 : MATLAB Function  TreatAsAtomicUnit=on
  Gain1 : Gain
  Gain2 : Gain  Gain=3
  Gain3 : Gain  Gain=Kir(:,1:2)  Multiplication=Matrix(K*u)
  Gain4 : Gain  Gain=Kir(3)
  Gain5 : Gain  Gain=0.8
  Gain6 : Gain  Gain=0.8
  Mux : Mux  Inputs=2
  Scope : Scope  NumInputPorts=2
  Sine Wave : dspsrcs4/Sine Wave  Amplitude=0.2*180/pi  Frequency=10  Phase=0  SampleMode=Discrete  OutComplex=Real  CompMethod=Trigonometric fcn  TableSize=Speed  SampleTime=0.02  SamplesPerFrame=1  ResetState=Restart at time zero  OutputFrames=off  dataType=double  wordLen=16  udDataType=sfix(16)  fracBitsMode=Best precision  numFracBits=15  OutDataTypeStr=double  LastOutDataTypeStr=double
  Sum : Sum  Inputs=---
  Sum1 : Sum  Inputs=|+-
  Sum2 : Sum  Inputs=|++
  Sum3 : Sum  Inputs=|+-
  Sum4 : Sum  Inputs=+|-
  Sum5 : Sum  Inputs=|+-
  Sum6 : Sum  Inputs=|++
  saturation : Saturate  UpperLimit=8.5  LowerLimit=-8.5
  dif_mode : Outport  VectorParamsAs1DForOutWhenUnconnected=off
  wires:
  Sum1/1 -> Gain4/1  "e"
  Sum4/1 -> Gain2/1  "sat"
  Gain3/1 -> Discrete derivative2/1(f)
  Gain2/1 -> Sum/1
  Mux/1 -> Gain3/1
  Sum/1 -> Discrete-Time Integrator/1  "u"
  Gain4/1 -> Sum/2
  Discrete derivative2/1(fdot) -> Sum/3
  Sum2/1 -> Sum4/1, saturation/1  "e"
  rudder/1 -> Gain/1
  v/1 -> Gain scheduling1/2(v)
  Gain scheduling1/1(Kr_s) -> Sum2/2
  Gain/1 -> Gain scheduling1/1(Kr)
  real_dif/1 -> Scope/2, Sum4/2
  Discrete-Time Integrator/1 -> Scope/1, Sum2/1, Gain scheduling/1(u)
  Sum3/1 -> Gain5/1  "e"
  roll/1 -> Sum5/2, Sum1/2, Mux/2
  Sum5/1 -> Gain6/1  "e"
  ref/1 -> Sum5/1, Sum1/1
  Gain6/1 -> Sum3/1
  saturation/1 -> dif_mode/1  "dif_val"
  P/1 -> Sum6/1
  Sum6/1 -> Mux/1

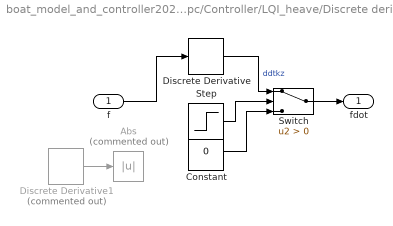
== system boat_model_and_controller2020mpc/Controller/LQI_heave/Discrete derivative1 ==
  f : Inport
  Abs : Abs  Commented=on
  Constant : Constant  Value=0
  Discrete Derivative : simulink/Discrete/Discrete Derivative  gainval=1.0  ICPrevScaledInput=0.0  OutMin=[]  OutMax=[]  OutDataType=fixdt(1, 16)  OutScaling=2^-10  DoSatur=off
  Discrete Derivative1 : simulink/Discrete/Discrete Derivative  Commented=on  gainval=1.0  ICPrevScaledInput=0.0  OutMin=[]  OutMax=[]  OutDataType=fixdt(1, 16)  OutScaling=2^-10  DoSatur=off
  Step : Step  Time=0.01  Before=-1
  Switch : Switch  Criteria=u2 > Threshold
  fdot : Outport  VectorParamsAs1DForOutWhenUnconnected=off
  wires:
  Switch/1 -> fdot/1
  f/1 -> Discrete Derivative/1
  Constant/1 -> Switch/3
  Discrete Derivative/1 -> Switch/1  "ddtkz"
  ? -> Discrete Derivative1/1
  Discrete Derivative1/1 -> Abs/1
  Step/1 -> Switch/2

== system boat_model_and_controller2020mpc/Controller/LQI_roll1/Discrete derivative2 ==
  f : Inport
  Constant : Constant  Value=0
  Discrete Derivative : simulink/Discrete/Discrete Derivative  gainval=1.0  ICPrevScaledInput=0.0  OutMin=[]  OutMax=[]  OutDataType=fixdt(1, 16)  OutScaling=2^-10  DoSatur=off
  Step : Step  Time=0.01  Before=-1
  Switch : Switch  Criteria=u2 > Threshold
  fdot : Outport  VectorParamsAs1DForOutWhenUnconnected=off
  wires:
  Discrete Derivative/1 -> Switch/1  "ddtkz"
  Constant/1 -> Switch/3
  Step/1 -> Switch/2
  f/1 -> Discrete Derivative/1
  Switch/1 -> fdot/1

== matlab function boat_model_and_controller2020mpc/Controller/LQI_roll1/Gain scheduling ==
  data: u input; u_s output; v input
function u_s = fcn(u,v)
v_ref = 6.4;
if(v>v_ref)
    u_s = u*v_ref^2/v^2;
else
    u_s = u;
end

== matlab function boat_model_and_controller2020mpc/BOAT/MATLAB Function ==
  data: u input; v input; Pitch_dot output; w input; Roll_dot output; Yaw_dot output; X_dot output; Y_dot output; Z_dot output; p input; q input; r input; Pitch input; Roll input; Yaw input
function [Pitch_dot,Roll_dot,Yaw_dot,X_dot,Y_dot,Z_dot] = kinematics(u,v,w,p,q,r,Pitch,Roll,Yaw)

%Inertial angular velocities
Yaw_dot = (q*sind(Roll)/(cosd(Roll)*cosd(Roll)*cosd(Pitch))+r/(cosd(Roll)*cosd(Pitch)))/(1+sind(Roll)*sind(Roll)/(cosd(Roll)*cosd(Roll)));
Pitch_dot = q/cosd(Roll) - Yaw_dot*cosd(Pitch)*sind(Roll)/cosd(Roll);
Roll_dot = p + Yaw_dot*sind(Pitch);


%Inertial to body axis matrix

R = [cosd(Pitch)*cosd(Yaw) cosd(Pitch)*sind(Yaw) -sind(Pitch);
        sind(Roll)*sind(Pitch)*cosd(Yaw)-cosd(Roll)*sind(Yaw) sind(Roll)*sind(Pitch)*sind(Yaw)+cosd(Roll)*cosd(Yaw) sind(Roll)*cosd(Pitch);
        cosd(Roll)*sind(Pitch)*cosd(Yaw)+sind(Roll)*sind(Yaw) cosd(Roll)*sind(Pitch)*sind(Yaw)-sind(Roll)*cosd(Yaw) cosd(Roll)*cosd(Pitch)];

%Inertial velocities

V_inertial = inv(R)*[u; v; w];
X_dot = V_inertial(1);
Y_dot = V_inertial(2);
Z_dot = V_inertial(3);
end

== matlab function boat_model_and_controller2020mpc/Controller/LQI_heave/Gain scheduling ==
  data: u input; u_s output; v input
function u_s = fcn(u,v)
v_ref = 6.4;
if(v>v_ref)
    u_s = u*v_ref^2/v^2;
else
    u_s = u;
end
